simulink model "DAddConMA_AM"  (Simulink 7.8)
settings: Solver=ode45  StartTime=0.0  StopTime=10.0  RelTol=1e-3
settings Model: Creator=fkolass  LastModifiedBy=fkolass

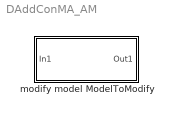
== system DAddConMA_AM ==
  modify model ModelToModify : Subsystem

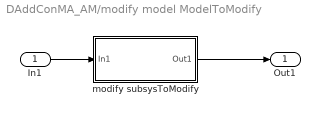
== system DAddConMA_AM/modify model ModelToModify ==
  In1 : Inport
  modify subsysToModify : Subsystem
  Out1 : Outport
  wires:
  In1/1 -> modify subsysToModify/1(In1)
  modify subsysToModify/1(Out1) -> Out1/1

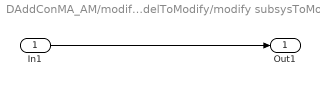
== system DAddConMA_AM/modify model ModelToModify/modify subsysToModify ==
  In1 : Inport
  Out1 : Outport
  wires:
  In1/1 -> Out1/1
